simulink model "Controller"  (R2024a)
settings: Solver=FixedStepDiscrete  StartTime=0.0  StopTime=10.0  FixedStep=0.01  RelTol=1e-3
model workspace (MATLAB code in the model file):
  | BodyParams;
  | ControlParams;
  | MotorParams;
  | WheelParams;
undefined symbols (not defined in the file): body_inertia, body_mass, Dinv, Dmat, motor_gyration, motor_resistance, nominal_voltage, pwm_limit, torque_limit, wheel_distance, wheel_radius
libraries: slpidlib x2, dspfdesign x1
settings Model: Creator=Marij  LastModifiedBy=Marij
settings OptimizationCC: DefaultParameterBehavior=Inlined  UseDivisionForNetSlopeComputation=on  GainParamInheritBuiltInType=on  UseFloatMulNetSlope=on  InlineInvariantSignals=on  PassReuseOutputArgsAs=Individual arguments  ZeroExternalMemoryAtStartup=off  ZeroInternalMemoryAtStartup=off  NoFixptDivByZeroProtection=on  EfficientFloat2IntCast=on  LifeSpan=1  OptimizeBlockOrder=speed  DifferentSizesBufferReuse=on  EfficientTunableParamExpr=on
settings DebuggingCC: ParameterTunabilityLossMsg=error
settings HardwareCC: ProdBitPerPointer=32  ProdBitPerSizeT=32  ProdBitPerPtrDiffT=32  ProdLargestAtomicInteger=Long  ProdLargestAtomicFloat=Double  ProdWordSize=32  ProdLongLongMode=on  ProdHWDeviceType=ARM Compatible->ARM Cortex-M
settings SFSimCC: MATLABDynamicMemAlloc=off
settings RTWCC: Description=Embedded Coder  SystemTargetFile=ert.tlc  GenCodeOnly=on  TemplateMakefile=ert_default_tmf
settings CodeAppCC: ForceParamTrailComments=on  IgnoreCustomStorageClasses=off  OperatorAnnotations=on  SimulinkDataObjDesc=on  SFDataObjDesc=on  CustomSymbolStrGlobalVar=rt$N$M  CustomSymbolStrType=$N$M  CustomSymbolStrFcn=$N$M$F  CustomSymbolStrMacro=$N$M  InsertBlockDesc=on
settings ERTTargetCC: TargetLangStandard=C99 (ISO)  GenerateSampleERTMain=on  IncludeMdlTerminateFcn=off  CombineSignalStateStructs=on  SuppressErrorStatus=on  SupportAbsoluteTime=off  SupportComplex=off  InlinedParameterPlacement=NonHierarchical  ERTCustomFileTemplate=example_file_process.tlc  ERTFilePackagingFormat=CompactWithDataFile

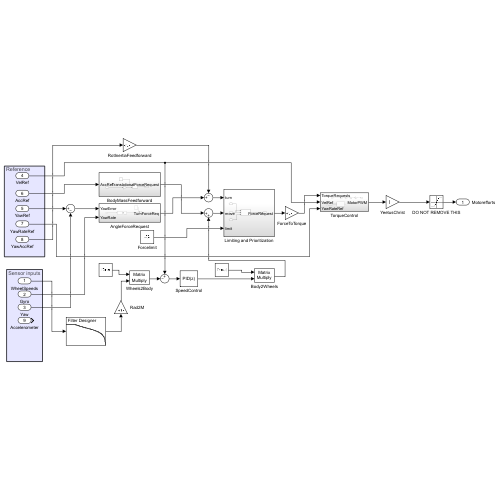
[thumbnail: Simulink's stored preview of the top-level diagram]
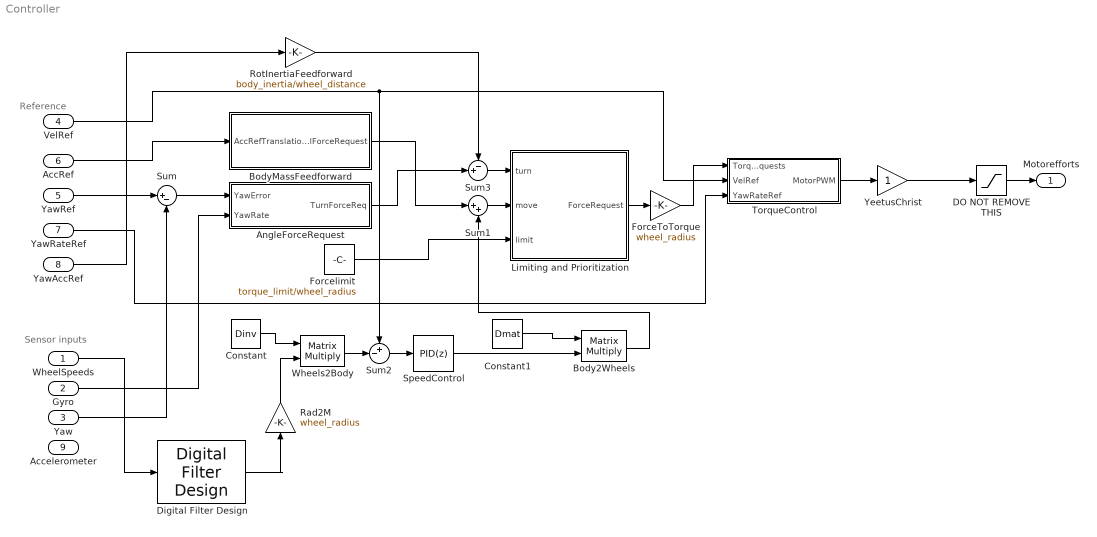
== system Controller ==
  note: Reference
  note: Sensor inputs
  WheelSpeeds : Inport  OutDataTypeStr=single  Unit=rad/s  PortDimensions=4  LockScale=on
  Gyro : Inport  Port=2  OutDataTypeStr=single  Unit=rad/s  PortDimensions=1
  Yaw : Inport  Port=3  OutDataTypeStr=single  Unit=rad  PortDimensions=1
  VelRef : Inport  Port=4  OutDataTypeStr=single  Unit=m/s  PortDimensions=2
  YawRef : Inport  Port=5
  AccRef : Inport  Port=6  OutDataTypeStr=single  Unit=m/s^2  PortDimensions=2
  YawRateRef : Inport  Port=7  OutDataTypeStr=single  Unit=rad/s
  YawAccRef : Inport  Port=8  OutDataTypeStr=single  Unit=rad/s^2
  Accelerometer : Inport  Port=9  OutDataTypeStr=single  Unit=m/s^2  PortDimensions=2
  AngleForceRequest : Subsystem
  Body2Wheels : Product  Multiplication=Matrix(*)
  BodyMassFeedforward : Subsystem
  Constant : Constant  Value=Dinv
  Constant1 : Constant  Value=Dmat
  DO NOT REMOVE THIS : Saturate  UpperLimit=pwm_limit  LowerLimit=-pwm_limit
  Digital Filter Design : dspfdesign/Digital Filter Design  mwdsp_browser_bugfix_var=off
  ForceToTorque : Gain  Gain=wheel_radius
  Forcelimit : Constant  Value=torque_limit/wheel_radius
  Limiting and Prioritization : Subsystem
  Rad2M : Gain  Gain=wheel_radius
  RotInertiaFeedforward : Gain  Gain=body_inertia/wheel_distance
  SpeedControl : slpidlib/PID Controller  Controller=PID  Form=Parallel  TimeDomain=Discrete-time  UseExternalTs=off  SampleTime=-1  IntegratorMethod=Forward Euler  FilterMethod=Forward Euler  ControllerParametersSource=internal  P=10  I=0  UseKiTs=off  D=0  UseExternalDerivativeSource=off  N=100  UseFilter=on  TunerSelectOption=Transfer Function Based (PID Tuner App)  InitialConditionSource=internal  InitialConditionForIntegrator=0  InitialConditionForFilter=0  DifferentiatorICPrevScaledInput=0  ExternalReset=none  TrackingMode=off  Kt=1  LimitOutput=off  SatLimitsSource=internal  UpperSaturationLimit=inf  LowerSaturationLimit=-inf  LinearizeAsGain=off  AntiWindupMode=none  Kb=1  LimitIntegrator=off  UpperIntegratorSaturationLimit=inf  LowerIntegratorSaturationLimit=-inf  POutMin=[]  POutMax=[]  IOutMin=[]  IOutMax=[]  DOutMin=[]  DOutMax=[]  NOutMin=[]  NOutMax=[]  SumOutMin=[]  SumOutMax=[]  SaturationOutMin=[]  SaturationOutMax=[]  PParamMin=[]  PParamMax=[]  IParamMin=[]  IParamMax=[]  DParamMin=[]  DParamMax=[]  NParamMin=[]  NParamMax=[]  KbParamMin=[]  KbParamMax=[]  KtParamMin=[]  KtParamMax=[]  KbOutMin=[]  KbOutMax=[]  KtOutMin=[]  KtOutMax=[]  IntegratorOutMin=[]  IntegratorOutMax=[]  FilterOutMin=[]  FilterOutMax=[]  SumI1OutMin=[]  SumI1OutMax=[]  SumI2OutMin=[]  SumI2OutMax=[]  SumI3OutMin=[]  SumI3OutMax=[]  SumI4OutMin=[]  SumI4OutMax=[]  SumDOutMin=[]  SumDOutMax=[]  DifferentiatorOutMin=[]  DifferentiatorOutMax=[]  FilterDiffOutCoefMin=[]  FilterDiffOutCoefMax=[]  ReciprocalOutMin=[]  ReciprocalOutMax=[]  SumDenOutMin=[]  SumDenOutMax=[]  SumNumOutMin=[]  SumNumOutMax=[]  DivideOutMin=[]  DivideOutMax=[]  UdiffTsProdOutMin=[]  UdiffTsProdOutMax=[]  NTsProdOutMin=[]  NTsProdOutMax=[]  UintegralTsProdOutMin=[]  UintegralTsProdOutMax=[]  UngainTsProdOutMin=[]  UngainTsProdOutMax=[]  ClampingZeroOutDataTypeStr=Inherit: Inherit via back propagation  ClampingZeroOutMin=[]  ClampingZeroOutMax=[]  FilterDenConstantOutDataTypeStr=Inherit: Inherit via back propagation  FilterDenConstantOutMin=[]  FilterDenConstantOutMax=[]  PCopyOutDataTypeStr=Inherit: Inherit via back propagation  PCopyOutMin=[]  PCopyOutMax=[]  NCopyOutDataTypeStr=Inherit: Inherit via back propagation  NCopyOutMin=[]  NCopyOutMax=[]  IntegratorContinuousStateAttributes=''  IntegratorStateMustResolveToSignalObject=off  IntegratorRTWStateStorageClass=Auto  FilterContinuousStateAttributes=''  FilterStateMustResolveToSignalObject=off  FilterRTWStateStorageClass=Auto  ParallelPVariant=InternalParameters  IdealPVariant=Disabled  IVariant=InternalParameters  DVariant=InternalParameters  IntegratorVariant=Discrete  SatVariant=Disabled  AWVariant=Passthrough  PCopyVariant=Disabled  TRVariant=Disabled  FdbkBlocksVariant=Forward  IdealPFdbkVariant=Disabled  SatFdbkVariant=Disabled  DerivativeFilterVariant=ForwardEulerFilter  NVariant=InternalParameters  NCopyVariant=Disabled  FilterICVariant=InternalICsFilter  IntegratorICVariant=InternalICs  ExternalResetVariant=Disabled  TRSumVariant=Passthrough  SumFdbkVariant=Disabled  SumVariant=Sum_PID  TsampFilterVariant=InternalTs  TsampNgainVariant=Passthrough  TsampIntegralVariant=Disabled_SignalSpec  ExternalSaturationOutDataTypeStr=Inherit: Same as second input  DerivativeSourceVariant=ErrorSignal
      settings: LibrarySourceBlock=simulink/Discrete/Discrete PID Controller
  Sum : Sum  Inputs=|+-
  Sum1 : Sum  Inputs=|++
  Sum2 : Sum  Inputs=+-|
  Sum3 : Sum  Inputs=-+|
  TorqueControl : Subsystem
  Wheels2Body : Product  Multiplication=Matrix(*)
  YeetusChrist : Gain
  Motorefforts : Outport  OutDataTypeStr=single  PortDimensions=4
  wires:
  YawRef/1 -> Sum/1
  Yaw/1 -> Sum/2
  Sum/1 -> AngleForceRequest/1(YawError)
  Gyro/1 -> AngleForceRequest/2(YawRate)
  AccRef/1 -> BodyMassFeedforward/1(AccRef)
  DO NOT REMOVE THIS/1 -> Motorefforts/1
  TorqueControl/1(MotorPWM) -> YeetusChrist/1
  ForceToTorque/1 -> TorqueControl/1(TorqueRequests)
  Forcelimit/1 -> Limiting and Prioritization/3(limit)
  Limiting and Prioritization/1(ForceRequest) -> ForceToTorque/1
  YeetusChrist/1 -> DO NOT REMOVE THIS/1
  VelRef/1 -> Sum2/1, TorqueControl/2(VelRef)
  YawRateRef/1 -> TorqueControl/3(YawRateRef)
  Constant/1 -> Wheels2Body/1
  BodyMassFeedforward/1(TranslationalForceRequest) -> Sum1/1
  Sum2/1 -> SpeedControl/1
  Sum1/1 -> Limiting and Prioritization/2(move)
  AngleForceRequest/1(TurnForceReq) -> Sum3/2
  Sum3/1 -> Limiting and Prioritization/1(turn)
  RotInertiaFeedforward/1 -> Sum3/1
  YawAccRef/1 -> RotInertiaFeedforward/1
  SpeedControl/1 -> Body2Wheels/2
  Constant1/1 -> Body2Wheels/1
  Body2Wheels/1 -> Sum1/2
  Wheels2Body/1 -> Sum2/2
  Digital Filter Design/1 -> Rad2M/1
  WheelSpeeds/1 -> Digital Filter Design/1
  Rad2M/1 -> Wheels2Body/2

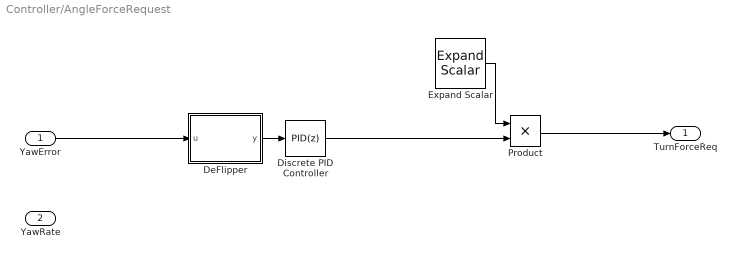
== system Controller/AngleForceRequest ==
  YawError : Inport  Unit=rad
  YawRate : Inport  Port=2
  DeFlipper : MATLAB Function  TreatAsAtomicUnit=on
  Discrete PID Controller : slpidlib/PID Controller  Controller=PID  Form=Parallel  TimeDomain=Discrete-time  UseExternalTs=off  SampleTime=-1  IntegratorMethod=Trapezoidal  FilterMethod=Trapezoidal  ControllerParametersSource=internal  P=3.0  I=0.0  UseKiTs=off  D=0.4  UseExternalDerivativeSource=off  N=100  UseFilter=on  TunerSelectOption=Transfer Function Based (PID Tuner App)  InitialConditionSource=internal  InitialConditionForIntegrator=0  InitialConditionForFilter=0  DifferentiatorICPrevScaledInput=0  ExternalReset=none  TrackingMode=off  Kt=1  LimitOutput=off  SatLimitsSource=internal  UpperSaturationLimit=inf  LowerSaturationLimit=-inf  LinearizeAsGain=off  AntiWindupMode=none  Kb=1  LimitIntegrator=off  UpperIntegratorSaturationLimit=inf  LowerIntegratorSaturationLimit=-inf  POutMin=[]  POutMax=[]  IOutMin=[]  IOutMax=[]  DOutMin=[]  DOutMax=[]  NOutMin=[]  NOutMax=[]  SumOutMin=[]  SumOutMax=[]  SaturationOutMin=[]  SaturationOutMax=[]  PParamMin=[]  PParamMax=[]  IParamMin=[]  IParamMax=[]  DParamMin=[]  DParamMax=[]  NParamMin=[]  NParamMax=[]  KbParamMin=[]  KbParamMax=[]  KtParamMin=[]  KtParamMax=[]  KbOutMin=[]  KbOutMax=[]  KtOutMin=[]  KtOutMax=[]  IntegratorOutMin=[]  IntegratorOutMax=[]  FilterOutMin=[]  FilterOutMax=[]  SumI1OutMin=[]  SumI1OutMax=[]  SumI2OutMin=[]  SumI2OutMax=[]  SumI3OutMin=[]  SumI3OutMax=[]  SumI4OutMin=[]  SumI4OutMax=[]  SumDOutMin=[]  SumDOutMax=[]  DifferentiatorOutMin=[]  DifferentiatorOutMax=[]  FilterDiffOutCoefMin=[]  FilterDiffOutCoefMax=[]  ReciprocalOutMin=[]  ReciprocalOutMax=[]  SumDenOutMin=[]  SumDenOutMax=[]  SumNumOutMin=[]  SumNumOutMax=[]  DivideOutMin=[]  DivideOutMax=[]  UdiffTsProdOutMin=[]  UdiffTsProdOutMax=[]  NTsProdOutMin=[]  NTsProdOutMax=[]  UintegralTsProdOutMin=[]  UintegralTsProdOutMax=[]  UngainTsProdOutMin=[]  UngainTsProdOutMax=[]  ClampingZeroOutDataTypeStr=Inherit: Inherit via back propagation  ClampingZeroOutMin=[]  ClampingZeroOutMax=[]  FilterDenConstantOutDataTypeStr=Inherit: Inherit via back propagation  FilterDenConstantOutMin=[]  FilterDenConstantOutMax=[]  PCopyOutDataTypeStr=Inherit: Inherit via back propagation  PCopyOutMin=[]  PCopyOutMax=[]  NCopyOutDataTypeStr=Inherit: Inherit via back propagation  NCopyOutMin=[]  NCopyOutMax=[]  IntegratorContinuousStateAttributes=''  IntegratorStateMustResolveToSignalObject=off  IntegratorRTWStateStorageClass=Auto  FilterContinuousStateAttributes=''  FilterStateMustResolveToSignalObject=off  FilterRTWStateStorageClass=Auto  ParallelPVariant=InternalParameters  IdealPVariant=Disabled  IVariant=InternalParameters  DVariant=InternalParameters  IntegratorVariant=Discrete  SatVariant=Disabled  AWVariant=Passthrough  PCopyVariant=Disabled  TRVariant=Disabled  FdbkBlocksVariant=Forward  IdealPFdbkVariant=Disabled  SatFdbkVariant=Disabled  DerivativeFilterVariant=TrapezoidalFilter  NVariant=InternalParameters  NCopyVariant=InternalParameters  FilterICVariant=InternalICsFilter  IntegratorICVariant=InternalICs  ExternalResetVariant=Disabled  TRSumVariant=Passthrough  SumFdbkVariant=Disabled  SumVariant=Sum_PID  TsampFilterVariant=InternalTs  TsampNgainVariant=Passthrough  TsampIntegralVariant=Disabled_SignalSpec  ExternalSaturationOutDataTypeStr=Inherit: Same as second input  DerivativeSourceVariant=ErrorSignal
      settings: LibrarySourceBlock=simulink/Discrete/Discrete PID Controller
  Expand Scalar : ExpandScalar  OutputDimensions=4  OutDataTypeStr=single  SampleTime=-1
  Product : Product  OutDataTypeStr=single
  TurnForceReq : Outport  Unit=N
  wires:
  Discrete PID Controller/1 -> Product/2
  Expand Scalar/1 -> Product/1
  Product/1 -> TurnForceReq/1
  YawError/1 -> DeFlipper/1(u)
  DeFlipper/1(y) -> Discrete PID Controller/1

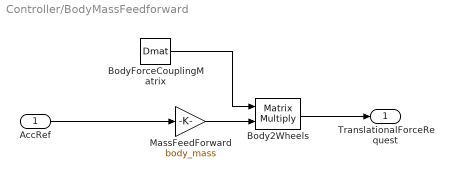
== system Controller/BodyMassFeedforward ==
  AccRef : Inport
  Body2Wheels : Product  Multiplication=Matrix(*)
  BodyForceCouplingMatrix : Constant  Value=Dmat  VectorParams1D=off  OutDataTypeStr=single
  MassFeedForward : Gain  Gain=body_mass
  TranslationalForceRequest : Outport  Unit=N
  wires:
  BodyForceCouplingMatrix/1 -> Body2Wheels/1
  MassFeedForward/1 -> Body2Wheels/2
  Body2Wheels/1 -> TranslationalForceRequest/1
  AccRef/1 -> MassFeedForward/1

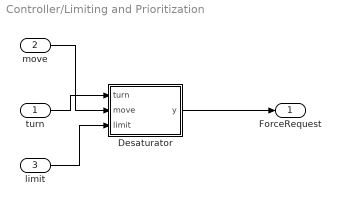
== system Controller/Limiting and Prioritization ==
  turn : Inport  Unit=N  PortDimensions=4
  move : Inport  Port=2  Unit=N  PortDimensions=4
  limit : Inport  Port=3  Unit=N
  Desaturator : MATLAB Function  TreatAsAtomicUnit=on
  ForceRequest : Outport  Unit=N  PortDimensions=4
  wires:
  turn/1 -> Desaturator/1(turn)
  move/1 -> Desaturator/2(move)
  limit/1 -> Desaturator/3(limit)
  Desaturator/1(y) -> ForceRequest/1

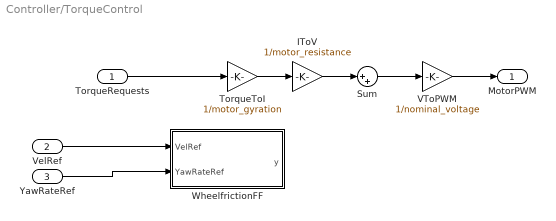
== system Controller/TorqueControl ==
  TorqueRequests : Inport
  VelRef : Inport  Port=2
  YawRateRef : Inport  Port=3
  IToV : Gain  Gain=1/motor_resistance
  Sum : Sum  Inputs=|++
  TorqueToI : Gain  Gain=1/motor_gyration
  VToPWM : Gain  Gain=1/nominal_voltage
  WheelfrictionFF : Subsystem
  MotorPWM : Outport
  wires:
  TorqueRequests/1 -> TorqueToI/1
  TorqueToI/1 -> IToV/1
  VToPWM/1 -> MotorPWM/1
  VelRef/1 -> WheelfrictionFF/1(VelRef)
  YawRateRef/1 -> WheelfrictionFF/2(YawRateRef)
  IToV/1 -> Sum/1
  Sum/1 -> VToPWM/1

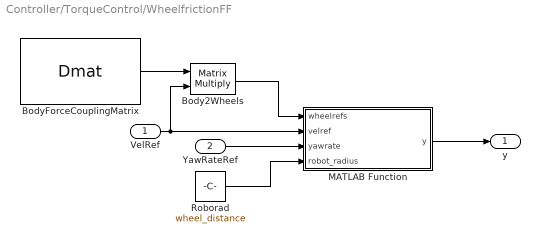
== system Controller/TorqueControl/WheelfrictionFF ==
  VelRef : Inport  PortDimensions=2
  YawRateRef : Inport  Port=2  PortDimensions=1
  Body2Wheels : Product  Multiplication=Matrix(*)
  BodyForceCouplingMatrix : Constant  Value=Dmat  VectorParams1D=off  OutDataTypeStr=single
  MATLAB Function : MATLAB Function  TreatAsAtomicUnit=on
  Roborad : Constant  Value=wheel_distance
  y : Outport  PortDimensions=4
  wires:
  BodyForceCouplingMatrix/1 -> Body2Wheels/1
  VelRef/1 -> MATLAB Function/2(velref), Body2Wheels/2
  Body2Wheels/1 -> MATLAB Function/1(wheelrefs)
  YawRateRef/1 -> MATLAB Function/3(yawrate)
  Roborad/1 -> MATLAB Function/4(robot_radius)
  MATLAB Function/1(y) -> y/1

== matlab function Controller/Limiting and Prioritization/Desaturator ==
  data: turn input; y output; move input; limit input
function y = fcn(turn, move, limit)
y = turn_prio_desaturator(turn, move, limit);
end

== matlab function Controller/AngleForceRequest/DeFlipper ==
  data: u input; y output
function y = fcn(u)

y = limit_angle(u);

== matlab function Controller/TorqueControl/WheelfrictionFF/MATLAB Function ==
  data: wheelrefs input; velref input; yawrate input; robot_radius input; y output
function y=fcn(wheelrefs, velref, yawrate, robot_radius)
[theta, rho] = cart2pol(velref(1), velref(2));
y = friction_feedforward(wheelrefs', rho, theta, yawrate, robot_radius)';
end
